simulink model "s1"  (R2013a)
settings: Solver=ode4  StartTime=0.0  StopTime=20.0  FixedStep=0.01  RelTol=1e-3
undefined symbols (not defined in the file): e0, e1, h, K, N, T
libraries: simulink x1
settings Model: Creator=adasdeb  LastModifiedBy=adasdeb
settings DataIOCC: LimitDataPoints=off

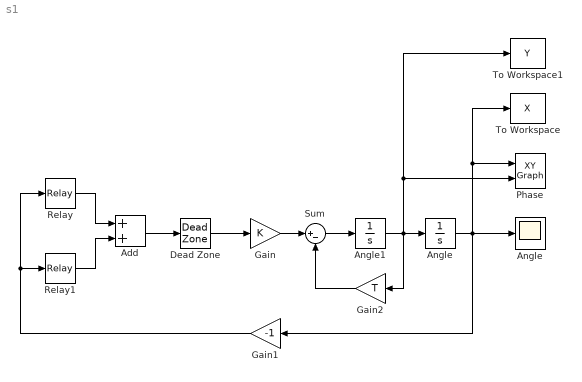
== system s1 ==
  Add : Sum
  Angle : Integrator  InitialCondition=e0
  "Angle " : Scope
  Angle1 : Integrator  InitialCondition=e1
  Dead Zone : DeadZone  LowerValue=-N  UpperValue=N  SaturateOnIntegerOverflow=on
  Gain : Gain  Gain=K
  Gain1 : Gain  Gain=-1
  Gain2 : Gain  Gain=T
  "Phase " : simulink/Sinks/XY Graph  xmin=-1  xmax=1  ymin=-1  ymax=1  st=-1
  Relay : Relay  OnSwitchValue=N+h  OffSwitchValue=N
  Relay1 : Relay  OnSwitchValue=-N  OffSwitchValue=-N-h  OnOutputValue=0  OffOutputValue=-1
  Sum : Sum  Inputs=|+-
  To Workspace : ToWorkspace  VariableName=X  SampleTime=-1
  To Workspace1 : ToWorkspace  VariableName=Y  SampleTime=-1
  wires:
  Relay/1 -> Add/1
  Relay1/1 -> Add/2
  Add/1 -> Dead Zone/1
  Dead Zone/1 -> Gain/1
  Gain1/1 -> Relay/1, Relay1/1
  Angle/1 -> "Angle "/1, To Workspace/1, "Phase "/1, Gain1/1
  Gain/1 -> Sum/1
  Sum/1 -> Angle1/1
  Angle1/1 -> To Workspace1/1, "Phase "/2, Angle/1, Gain2/1
  Gain2/1 -> Sum/2
